simulink model "untitled"  (R2018a)
settings: Solver=VariableStepAuto  StartTime=0.0  StopTime=1  RelTol=1e-3
values from neighbouring files (symbols this model uses):
  Cf = 1 / (wn * Xf)    (= 0.000159154943092)    [SequenceSeparation_script.m]
  Lr = Vdc / (0.8 * 2^0.5 * ( Sn / 3^0.5 / Vrms) * Fsw)    (= 0.001)    [SequenceSeparation_script.m]
  Rf = 1 / ( 3 * 2 * pi * fres * Cf)    [SequenceSeparation_script.m]
  Rr = 0.005    [SequenceSeparation_script.m]
  Ts = 1e-6    (= 1e-06)    [SequenceSeparation_script.m]
  Ts_pwm = 1/200000    (= 5e-06)    [SequenceSeparation_script.m]
  Vdc = 2    [SequenceSeparation_script.m]
libraries: powerlib x36, pwrsysVSrc_202301 x2, powerlib_meascontrol x1
settings Model: Creator=daniemot  LastModifiedBy=daniemot

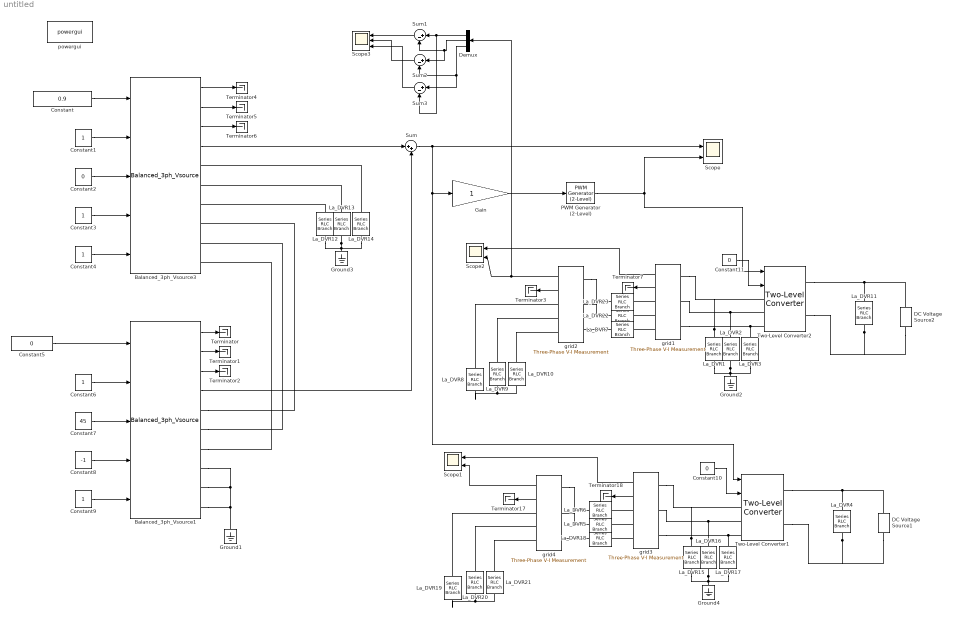
== system untitled ==
  Balanced_3ph_Vsource1 : pwrsysVSrc_202301/Balanced_3ph_Vsource  BaseAmp=1  fn=50  AmpIni=1  SeqIni=1  AngIni=0  FIni=50  HarmIni=1
  Balanced_3ph_Vsource3 : pwrsysVSrc_202301/Balanced_3ph_Vsource  BaseAmp=1  fn=50  AmpIni=1  SeqIni=1  AngIni=0  FIni=50  HarmIni=1
  Constant : Constant  Value=0.9
  Constant{1,3..4,6,9} (5 alike) : Constant
  Constant{2,5,10..11} (4 alike) : Constant  Value=0
  Constant7 : Constant  Value=45
  Constant8 : Constant  Value=-1
  DC Voltage Source1 : powerlib/Electrical Sources/DC Voltage Source  Amplitude=Vdc  Measurements=None
  DC Voltage Source2 : powerlib/Electrical Sources/DC Voltage Source  Amplitude=Vdc  Measurements=None
  Demux : Demux  Outputs=3
  Gain : Gain
  Ground{1..4} (4 alike) : powerlib/Elements/Ground  LConnTagsString=a
  La_DVR{1..3,12..17} (9 alike) : powerlib/Elements/Series RLC Branch  LConnTagsString=__new0  RConnTagsString=__new0  BranchType=R  Resistance=1e6  Inductance=0.3/(2*pi*50)  SetiL0=off  InitialCurrent=0  Capacitance=1.0  Setx0=off  InitialVoltage=0  Measurements=None
  La_DVR{8..10,19..21} (6 alike) : powerlib/Elements/Series RLC Branch  LConnTagsString=__new0  RConnTagsString=__new0  BranchType=RC  Resistance=Rf  Inductance=0.3/(2*pi*50)  SetiL0=off  InitialCurrent=0  Capacitance=Cf  Setx0=off  InitialVoltage=0  Measurements=None
  La_DVR11 : powerlib/Elements/Series RLC Branch  LConnTagsString=__new0  RConnTagsString=__new0  BranchType=R  Resistance=100000  Inductance=0.3/(2*pi*50)  SetiL0=off  InitialCurrent=0  Capacitance=Cf  Setx0=off  InitialVoltage=0  Measurements=None
  La_DVR{5..7,18,22..23} (6 alike) : powerlib/Elements/Series RLC Branch  LConnTagsString=__new0  RConnTagsString=__new0  BranchType=RL  Resistance=Rr  Inductance=Lr  SetiL0=off  InitialCurrent=0  Capacitance=1.0  Setx0=off  InitialVoltage=0  Measurements=None
  La_DVR4 : powerlib/Elements/Series RLC Branch  LConnTagsString=__new0  RConnTagsString=__new0  BranchType=R  Resistance=100000  Inductance=0.3/(2*pi*50)  SetiL0=off  InitialCurrent=0  Capacitance=Cf  Setx0=off  InitialVoltage=0  Measurements=None
  PWM Generator (2-Level) : powerlib_meascontrol/Pulse & Signal Generators/PWM Generator (2-Level)  ModulatorType=Three-phase bridge (6 pulses)  ModulatorMode=Unsynchronized  Fc=Fsw  Pc=90  nF=27  MinMax="[ -1  1 ]"  SamplingTechnique=Asymmetrical regular (double edge)  ModulatingSignals=off  m=0.8  Freq=60  Phase=0  Ts=Ts_pwm  ShowCarrierOutport=off
      settings: SourceProductName=Simscape Power Systems
  Scope : Scope  NumInputPorts=2
  Scope1 : Scope  NumInputPorts=2
  Scope2 : Scope  NumInputPorts=2
  Scope3 : Scope  NumInputPorts=3
  Sum : Sum  Inputs=|++
  Sum1 : Sum  Inputs=|+-
  Sum2 : Sum  Inputs=|+-
  Sum3 : Sum  Inputs=|+-
  Terminator{,1..7,17..18} (10 alike) : Terminator
  Two-Level Converter1 : powerlib/Power Electronics/Two-Level Converter  ModelType=Average model (Uref-controlled)  Ron=0.00001  Rs=1e6  Cs=inf  Vforward=[0,0]  Ron_Diode=0.001e-3  Rs_Diode=1e6  Cs_Diode=inf  Vf_Diode=1e-6  Rs_CurrentSource=inf
      settings: SourceProductName=Simscape Power Systems  SourceProductBaseCode=PS
  Two-Level Converter2 : powerlib/Power Electronics/Two-Level Converter  ModelType=Switching devices  Ron=0.00001  Rs=1e6  Cs=inf  Vforward=[0,0]  Ron_Diode=0.001e-3  Rs_Diode=1e6  Cs_Diode=inf  Vf_Diode=1e-6  Rs_CurrentSource=inf
      settings: SourceProductName=Simscape Power Systems  SourceProductBaseCode=PS
  grid{1..4} (4 alike) : powerlib/Measurements/Three-Phase V-I Measurement  VoltageMeasurement=phase-to-ground  SetLabelV=off  LabelV=vgrid  Vpu=off  VpuLL=off  CurrentMeasurement=yes  SetLabelI=off  LabelI=igrid  Ipu=off  Pbase=sn  Vbase=uab  OutputType=Complex  PhasorSimulation=off  PSBequivalent=0
  powergui : powerlib/powergui  Priority=1  SimulationMode=Discrete  SampleTime=Ts  frequency=60  Iterations=50  frequencyindice=0  Pbase=100e6  ErrMax=1e-4  UnitsV=kV  UnitsW=MW  buscounter=0  FunctionMessages=off  echomessages=off  EnableUseOfTLC=off  CurrentSourceSwitches=off  DisableSnubberDevices=off  DisableRonSwitches=off  DisableVfSwitches=off  DisplayEquations=off  SolverType=Tustin/Backward Euler (TBE)  Interpol=off  ExternalGateDelay=off  methode=off  Ts=100  x0status=blocks  SPID=off  SwTol=0  HookPort=off  RestoreLinks=warning  ResistiveCurrentMeasurement=off  Frange=[60:1:1600]  Ylog=on  Xlog=on  ShowGrid=on  save=off  variable=ZData  structure=0  ZoomFFT=off  StartTime=0.0  cycles=1  DisplayStyle=1  fundamental=60  FreqAxis=off  MaxFrequency=1000  frequencyindicesteady=1  RmsSteady=1  display=off
  wires:
  Balanced_3ph_Vsource3/2 -> Terminator5/1
  Constant9/1 -> Balanced_3ph_Vsource1/5
  Constant8/1 -> Balanced_3ph_Vsource1/4
  Balanced_3ph_Vsource3/1 -> Terminator4/1
  Constant/1 -> Balanced_3ph_Vsource3/1
  Balanced_3ph_Vsource1/2 -> Terminator1/1
  Balanced_3ph_Vsource3/3 -> Terminator6/1
  Balanced_3ph_Vsource1/1 -> Terminator/1
  Constant6/1 -> Balanced_3ph_Vsource1/2
  Constant1/1 -> Balanced_3ph_Vsource3/2
  Constant3/1 -> Balanced_3ph_Vsource3/4
  Constant4/1 -> Balanced_3ph_Vsource3/5
  Constant2/1 -> Balanced_3ph_Vsource3/3
  Balanced_3ph_Vsource1/3 -> Terminator2/1
  Constant7/1 -> Balanced_3ph_Vsource1/3
  Balanced_3ph_Vsource3/4 -> Sum/1
  Balanced_3ph_Vsource1/4 -> Sum/2
  Constant5/1 -> Balanced_3ph_Vsource1/1
  PWM Generator (2-Level)/1 -> Scope/2, Two-Level Converter2/1
  Constant10/1 -> Two-Level Converter1/2
  grid3/1 -> Scope1/1
  grid4/2 -> Terminator17/1
  grid4/1 -> Scope1/2
  grid3/2 -> Terminator18/1
  Sum/1 -> Two-Level Converter1/1, Gain/1, Scope/1
  grid1/1 -> Scope2/1
  Constant11/1 -> Two-Level Converter2/2
  grid1/2 -> Terminator7/1
  grid2/2 -> Terminator3/1
  grid2/1 -> Demux/1, Scope2/2
  Gain/1 -> PWM Generator (2-Level)/1
  Demux/1 -> Sum3/2, Sum1/1
  Demux/2 -> Sum2/1, Sum1/2
  Demux/3 -> Sum3/1, Sum2/2
  Sum1/1 -> Scope3/1
  Sum2/1 -> Scope3/2
  Sum3/1 -> Scope3/3
  connections:
  Balanced_3ph_Vsource1/RConn4 -- Ground1/LConn1 -- Balanced_3ph_Vsource1/RConn6 -- Balanced_3ph_Vsource1/RConn5
  Balanced_3ph_Vsource1/RConn2 -- Balanced_3ph_Vsource3/RConn5
  Balanced_3ph_Vsource1/RConn3 -- Balanced_3ph_Vsource3/RConn6
  Balanced_3ph_Vsource1/RConn1 -- Balanced_3ph_Vsource3/RConn4
  Ground3/LConn1 -- La_DVR13/LConn1 -- La_DVR12/LConn1 -- La_DVR14/LConn1
  La_DVR12/RConn1 -- Balanced_3ph_Vsource3/RConn3
  La_DVR13/RConn1 -- Balanced_3ph_Vsource3/RConn2
  La_DVR14/RConn1 -- Balanced_3ph_Vsource3/RConn1
  La_DVR20/LConn1 -- La_DVR19/LConn1 -- La_DVR21/LConn1
  Ground4/LConn1 -- La_DVR16/LConn1 -- La_DVR15/LConn1 -- La_DVR17/LConn1
  Two-Level Converter1/LConn2 -- grid3/LConn2 -- La_DVR16/RConn1
  Two-Level Converter1/LConn3 -- grid3/LConn3 -- La_DVR17/RConn1
  La_DVR15/RConn1 -- Two-Level Converter1/LConn1 -- grid3/LConn1
  La_DVR4/RConn1 -- DC Voltage Source1/LConn1 -- Two-Level Converter1/RConn2
  Two-Level Converter1/RConn1 -- DC Voltage Source1/RConn1 -- La_DVR4/LConn1
  grid4/RConn2 -- La_DVR20/RConn1
  grid4/RConn3 -- La_DVR21/RConn1
  grid3/RConn3 -- La_DVR18/LConn1
  grid3/RConn2 -- La_DVR5/LConn1
  grid4/LConn3 -- La_DVR18/RConn1
  grid4/LConn2 -- La_DVR5/RConn1
  grid4/LConn1 -- La_DVR6/RConn1
  grid3/RConn1 -- La_DVR6/LConn1
  La_DVR19/RConn1 -- grid4/RConn1
  Two-Level Converter2/LConn3 -- grid1/LConn3 -- La_DVR3/RConn1
  Two-Level Converter2/LConn2 -- grid1/LConn2 -- La_DVR2/RConn1
  La_DVR1/RConn1 -- Two-Level Converter2/LConn1 -- grid1/LConn1
  Two-Level Converter2/RConn1 -- DC Voltage Source2/RConn1 -- La_DVR11/LConn1
  La_DVR11/RConn1 -- DC Voltage Source2/LConn1 -- Two-Level Converter2/RConn2
  La_DVR9/LConn1 -- La_DVR8/LConn1 -- La_DVR10/LConn1
  Ground2/LConn1 -- La_DVR2/LConn1 -- La_DVR1/LConn1 -- La_DVR3/LConn1
  grid1/RConn3 -- La_DVR7/LConn1
  La_DVR8/RConn1 -- grid2/RConn1
  grid1/RConn1 -- La_DVR23/LConn1
  grid2/LConn1 -- La_DVR23/RConn1
  grid1/RConn2 -- La_DVR22/LConn1
  grid2/RConn3 -- La_DVR10/RConn1
  grid2/RConn2 -- La_DVR9/RConn1
  grid2/LConn3 -- La_DVR7/RConn1
  grid2/LConn2 -- La_DVR22/RConn1
